simulink model "VFlexP"  (R2025a)
settings: Solver=ode23tb  StartTime=0.0  StopTime=40  FixedStep=5e-5
model workspace (MAT data in the model file):
  DCop_DCBUCK : object (value not decoded)
  Grid_CCVSC_idx = [2; 3; 4; 5; 6; 7; 8; 9; 10; 11; 12]
  Grid_CCVSCs = 1
  Grid_CCVSCs_buses = 1
  Grid_CCVSCs_toM = [0 1 0 0 0 0 0 0 0 0 0 0 ... (781 elements, 71x11)]
  Grid_C_Lines = [0.1 0.1 0.1 0.1]
  Grid_Cbuses = [0.05000002 0.10000002 0.10000002 0.10000002 0.05000002]
  Grid_DC : object (value not decoded)
  Grid_DCop_DCBUCK : object (value not decoded)
  Grid_DCop_DC_PES : object (value not decoded)
  Grid_DFIGs = 1
  Grid_DFIGs_buses = 1
  Grid_DGs : string (value not decoded)
  Grid_From_buses = [1 2 4 4]
  Grid_GFls = 1
  Grid_GFls_buses = 1
  Grid_GFr_idx = [1; 2; 3]
  Grid_GFrs = 1
  Grid_GFrs_buses = 1
  Grid_GFrs_toM = [1 0 0 0 0 0 0 0 0 1 0 0 ... (15 elements, 5x3)]
  Grid_IG_idx = 1
  Grid_IGs = 1
  Grid_IGs_buses = 1
  Grid_IGs_toM = [1; 0]
  Grid_L_Lines = [0.5 0.5 0.5 0.5]
  Grid_L_Loads = [0.000959999944704 0.000156249997559 0.00154855477548]
  Grid_Lines_fromM : object (value not decoded)
  Grid_Lines_toM : object (value not decoded)
  Grid_Load_buses = [2; 3; 4]
  Grid_Load_busesDC = []
  Grid_MGES_idx = [1; 2; 3]
  Grid_MGESs = 1
  Grid_MGESs_buses = [1; 5; 3]
  Grid_MGESs_toM = [1 0 0 0 0 0 0 0 0 1 0 0 ... (15 elements, 5x3)]
  Grid_MSGs = 1
  Grid_MSGs_buses = 1
  Grid_Nbuses = 5
  Grid_PQ_gen = [3; 2; 2]
  Grid_Ploads = [1250 4000 1250]
  Grid_PloadsDC = []
  Grid_Ps_lf = [0.274439537683 0.78 0.3]
  Grid_Qloads = [0.3 0.5 0.5]
  Grid_Qs_lf = [-0.0366071562958 0.126505596722 -0.0162964024532]
  Grid_R_Lines = [0.01 0.01 0.01 0.01]
  Grid_R_Loads = [3.9999997696 1.24999998047 3.8713869387]
  Grid_R_Loads_DC = 0
  Grid_Rcf = [50000000 50000000 50000000 50000000 50000000]
  Grid_SCs = 1
  Grid_SCs_buses = 1
  Grid_SG_idx = 1
  Grid_SGs = 1
  Grid_SGs_buses = 1
  Grid_SGs_toM = [1; 0]
  Grid_To_buses = [2 3 3 5]
  Grid_VCVSC_idx = [1; 2; 3; 4; 5; 6; 7; 8; 9; 10; 11; 12]
  Grid_VCVSCs = 1
  Grid_VCVSCs_buses = [1; 2; 3; 6; 8; 9; 12; 58; 59; 60; 63; 65]
  Grid_VCVSCs_toM = [1 0 0 0 0 0 0 0 0 0 0 0 ... (852 elements, 71x12)]
  Grid_VSM_idx = [1; 2; 3]
  Grid_VSMs = 1
  Grid_VSMs_buses = 1
  Grid_VSMs_toM = [1 0 0 0 0 0 0 0 0 1 0 0 ... (15 elements, 5x3)]
  Grid_admitt_matrix = [2.15353135314-19.7953135314i  -1.9801980198+19.801980198i; -1.9801980198+19.801980198i  2.15353135314-19.7953135314i]
  Grid_admitt_matrix_noloads = [1.98686468647-19.7953135314i  -1.9801980198+19.801980198i; -1.9801980198+19.801980198i  1.98686468647-19.7953135314i]
  Grid_bus = [1; 2; 6; 7; 8]
  Grid_busDC_complexity = [1 1 1]
  Grid_busDC_complexity_PF = [2 2 2]
  Grid_bus_complexity = [1 1 1 1 1]
  Grid_bus_complexity_PF = [1 1 1 1 1]
  Grid_buses_lf = [1; 5; 3]
  Grid_conductance_matrix = [100.00000002  -100  0; -100  200.00000002  -100; 0  -100  100.00000002]
  Grid_conductance_matrix_noloads = [100.00000002  -100  0; -100  200.00000002  -100; 0  -100  100.00000002]
  Grid_fref : object (value not decoded)
  Grid_gen_static_params : mBase (value not decoded)
  Grid_iPs_lf = [3.64378984326 1.28205128205 3.33333333333]
  Grid_iQs_lf = [-27.3170631425 7.90478860943 -61.3632366329]
  Grid_iadmitt_matrix = [2.88165849328-0.0982918688642i  2.87905051706-0.123273862303i; 2.87905051706-0.123273862303i  2.88165849328-0.0982918688642i]
  Grid_iadmitt_matrix_noloads = [37.5012524798-37.4874983544i  37.4987475202-37.5125016456i; 37.4987475202-37.5125016456i  37.5012524798-37.4874983544i]
  Grid_iconductance_matrix = [16666671.4556  16666671.4489  16666671.4456; 16666671.4489  16666671.4522  16666671.4489; 16666671.4456  16666671.4489  16666671.4556]
  Grid_iconductance_matrix_noloads = [16666671.4556  16666671.4489  16666671.4456; 16666671.4489  16666671.4522  16666671.4489; 16666671.4456  16666671.4489  16666671.4556]
  Grid_init_OK_bool = 1
  Grid_intconv_PF : object (value not decoded)
  Grid_lf_op : op_report (value not decoded)
  Grid_lineDC_complexity = [1 1]
  Grid_lineDC_complexity_PF = [2 2]
  Grid_line_complexity = [1 1 1 1]
  Grid_line_complexity_PF = [3 3 3 3]
  Grid_loadDC_complexity = []
  Grid_loadDC_complexity_PF = []
  Grid_load_complexity = [3 3 3]
  Grid_load_complexity_PF = [4 4 4]
  Grid_opDC_CCVSC : object (value not decoded)
  Grid_opDC_VSM : object (value not decoded)
  Grid_opGFr : object (value not decoded)
  Grid_opVCVSC : object (value not decoded)
  Grid_op_CCVSC : object (value not decoded)
  Grid_op_IG : object (value not decoded)
  Grid_op_MGES : object (value not decoded)
  Grid_op_SG : object (value not decoded)
  Grid_op_VSM : object (value not decoded)
  Grid_shift_lines = [0 0 0 0]
  Grid_tap_lines = [1 1 1 1]
  Grid_v_buses_mod = [1 1 1 0.9837920967 1]
  LinsysParamChangeStruct : Param1 (value not decoded)
  Lline = 0.01
  Rline = 1e-05
  linsys : object (value not decoded)
symbols that are objects in the model workspace (value not decoded): Grid_DCop_DC_PES, Grid_DCop_DCBUCK, Grid_op_CCVSC, Grid_op_IG, Grid_op_MGES, Grid_op_SG, Grid_op_VSM, Grid_opDC_CCVSC, Grid_opDC_VSM, Grid_opGFr, Grid_opVCVSC
undefined symbols (not defined in the file): block_buses_DC, block_idx, CCVSC_idx, Cf, costs, costs2, D, DFIGs_nodes, DiscIntNeverNeededParam, entity, Fb, Fi, From_nodes, grid_linsys, Grid_op_DFIG, Grid_op_DFIG_PQ, Grid_op_MSG, Grid_op_SC, Grid_op_VCVSC, H, initial_states_grid, K_1, K_3, K_5, K_A, K_C, K_IM, K_IR, K_P, K_PM, K_PR, K_S1, K_S2, K_S3, Ki_w, Kic, Kiv, Kp_id, Kp_theta, Kp_w, Kpc, Kpv, last_send, Lc, Lf, Lfd, Lkd1, Lkd2, Lkq1, Lkq2, Lkq3, Lmd, Lmq, Lsd, Lsq, m, M, Matrix_flux_to_i, mp, MSGs_buses ... (+44)
libraries: simulink x1048, eeGeneralControl x12
(part 10 of 50)

== system VFlexP/Grid/Generators/DFIG/w_ref_TF ==
  in : Inport
  Gain : Gain  Gain=1/T_s
  Sum4 : Sum  Inputs=|+-
  x_a : Integrator  InitialCondition=Grid_op_DFIG.op.States(23).x'
  out : Outport
  wires:
  Gain/1 -> x_a/1
  Sum4/1 -> Gain/1
  x_a/1 -> out/1, Sum4/2
  in/1 -> Sum4/1

== system VFlexP/Grid/Generators/GFl/CC ==
  note: 1) Add Subsystem or Model blocks as valid variant choices.
      | 2) You cannot connect blocks at this level. At simulation, connectivity is automatically
      | determined, based on the active variant and port name matching.
  idref : Inport
  iqref : Inport  Port=2
  vod : Inport  Port=3
  voq : Inport  Port=4
  omega : Inport  Port=5
  dynamic : Subsystem  VariantControl=dynamic  mask{dynamic_line=Dynamic}
      mask prompts: dynamic_line "Line"
      mask TypeOptions dynamic_line: RL/dynamic
  static : Subsystem  VariantControl=static
  idiref : Outport
  iqiref : Outport  Port=2

== system VFlexP/Grid/Generators/GFl/For Each Subsystem ==
  In1 : Inport  Partition=on  PartitionDimension=1  PartitionWidth=1  PartitionOffset=0
  For Each : ForEach  DisableCoverage=on
  State-Space : StateSpace  A=[]  B=[]  C=[]  D=block_toM  InitialCondition=0  ParameterTunability=Optimized
  Transpose : Math  Operator=transpose
  Transpose1 : Math  Operator=transpose
  Out1 : Outport  ConcatenationDimension=1
  wires:
  Transpose1/1 -> Out1/1
  In1/1 -> Transpose/1
  Transpose/1 -> State-Space/1
  State-Space/1 -> Transpose1/1

== system VFlexP/Grid/Generators/GFl/LPF ==
  In1 : Inport
  Gain : Gain  Gain=1e2
  I : Integrator  InitialCondition=Grid_op_CCVSC.op.States(1).x'
  Sum4 : Sum  Inputs=|+-
  Out1 : Outport
  wires:
  Gain/1 -> I/1
  Sum4/1 -> Gain/1
  In1/1 -> Sum4/1
  I/1 -> Out1/1, Sum4/2

== system VFlexP/Grid/Generators/GFl/LPF1 ==
  In1 : Inport
  Gain : Gain  Gain=1e2
  I : Integrator  InitialCondition=Grid_op_CCVSC.op.States(2).x'
  Sum4 : Sum  Inputs=|+-
  Out1 : Outport
  wires:
  I/1 -> Sum4/2, Out1/1
  In1/1 -> Sum4/1
  Sum4/1 -> Gain/1
  Gain/1 -> I/1

== system VFlexP/Grid/Generators/GFl/LPF2 ==
  In1 : Inport
  Gain : Gain  Gain=1e2
  I : Integrator  InitialCondition=Grid_op_CCVSC.op.States(3).x'
  Sum4 : Sum  Inputs=|+-
  Out1 : Outport
  wires:
  Gain/1 -> I/1
  Sum4/1 -> Gain/1
  In1/1 -> Sum4/1
  I/1 -> Out1/1, Sum4/2

== system VFlexP/Grid/Generators/GFl/LPF3 ==
  In1 : Inport
  Gain : Gain  Gain=1e2
  I : Integrator  InitialCondition=Grid_op_CCVSC.op.States(4).x'
  Sum4 : Sum  Inputs=|+-
  Out1 : Outport
  wires:
  I/1 -> Sum4/2, Out1/1
  In1/1 -> Sum4/1
  Sum4/1 -> Gain/1
  Gain/1 -> I/1

== system VFlexP/Grid/Generators/GFl/LPF_d ==
  In1 : Inport
  Gain : Gain  Gain=iTf
  I : Integrator  InitialCondition=Grid_op_CCVSC.op.States(5).x'
  Sum4 : Sum  Inputs=|+-
  Out1 : Outport
  wires:
  I/1 -> Sum4/2, Out1/1
  In1/1 -> Sum4/1
  Sum4/1 -> Gain/1
  Gain/1 -> I/1

== system VFlexP/Grid/Generators/GFl/LPF_q ==
  In1 : Inport
  Gain : Gain  Gain=iTf
  I : Integrator  InitialCondition=Grid_op_CCVSC.op.States(6).x'
  Sum4 : Sum  Inputs=|+-
  Out1 : Outport
  wires:
  Sum4/1 -> Gain/1
  In1/1 -> Sum4/1
  I/1 -> Sum4/2, Out1/1
  Gain/1 -> I/1

== system VFlexP/Grid/Generators/GFl/PC ==
  vodi : Inport
  voq : Inport  Port=2
  vodi1 : Inport  Port=3
  vodi2 : Inport  Port=4
  omega : Inport  Port=5
  Constant : Constant
  Constant1 : Constant  Value=Eref  VectorParams1D=off
  Constant2 : Constant  Value=Inf
  Divide : Product  Inputs=*/
  Divide1 : Product  Inputs=*/
  Gain1 : Gain  Gain=alphaqcoef
  Gain2 : Gain  Gain=alphapcoef
  LPF_d : Subsystem  Commented=through
  LPF_q : Subsystem  Commented=through
  Product{,1..5} (6 alike) : Product
  Saturation : Subsystem  Commented=through
  Sum : Sum  Inputs=|++
  Sum1 : Sum  Inputs=|+-
  Sum3 : Sum  Inputs=|-+
  Sum4 : Sum  Inputs=|++
  Sum5 : Sum  Inputs=++|
  Sum6 : Sum  Inputs=|-+
  Sum7 : Sum  Inputs=++|
  Switch : Switch  Criteria=u2 > Threshold  Threshold=1e-5  ZeroCross=off  SaturateOnIntegerOverflow=off  InputSameDT=off
  Output : Outport
  Output1 : Outport  Port=2
  wires:
  LPF_q/1(Out1) -> Product5/1, Product5/2, Product2/2, Product1/1
  LPF_d/1(Out1) -> Product4/1, Product4/2, Product/2, Product3/2, Sum6/1
  Switch/1 -> Divide1/2, Divide/2
  Constant2/1 -> Switch/3
  vodi2/1 -> Sum7/2  "Qref"
  Sum6/1 -> Gain1/1
  omega/1 -> Sum3/1  "omega"
  Gain1/1 -> Sum7/1
  Constant1/1 -> Sum6/2
  vodi1/1 -> Sum5/2  "Pref"
  Gain2/1 -> Sum5/1
  Constant/1 -> Sum3/2
  Sum3/1 -> Gain2/1
  Sum/1 -> Divide/1
  Sum4/1 -> Switch/1, Switch/2
  Sum1/1 -> Divide1/1
  Sum5/1 -> Product/1, Product2/1  "Prefnew"
  Product5/1 -> Sum4/2
  Product4/1 -> Sum4/1
  voq/1 -> LPF_q/1(In1)  "voq"
  vodi/1 -> LPF_d/1(In1)  "vod"
  Sum7/1 -> Product3/1, Product1/2  "Qrefnew"
  Product3/1 -> Sum1/2
  Product2/1 -> Sum1/1
  Product1/1 -> Sum/2
  Product/1 -> Sum/1
  Divide/1 -> Saturation/1(ildref)  "ildref"
  Divide1/1 -> Saturation/2(ilqref)  "ilqref"
  Saturation/1(y) -> Output/1
  Saturation/2(y1) -> Output1/1

== system VFlexP/Grid/Generators/GFl/PLL ==
  note: 1) Add Subsystem or Model blocks as valid variant choices.
      | 2) You cannot connect blocks at this level. At simulation, connectivity is automatically
      | determined, based on the active variant and port name matching.
  voutangle : Inport
  vq : Inport  Port=2
  omega : Inport  Port=3
  dynamic : Subsystem  VariantControl=dynamic
  static : Subsystem  VariantControl=static
  theta : Outport
  omega_point : Outport  Port=2

== system VFlexP/Grid/Generators/GFl/Reference frame transform3 ==
  in_d : Inport
  theta : Inport  Port=2
  in_q : Inport  Port=3
  Complex to Real-Imag : ComplexToRealImag
  Cos : Trigonometry  SCDEnableBlockLinearizationSpecification=on  Operator=cos
  Product : Product
  Real-Imag to Complex : RealImagToComplex
  Real-Imag to Complex1 : RealImagToComplex
  Sin : Trigonometry  SCDEnableBlockLinearizationSpecification=on
  out_d : Outport
  out_q : Outport  Port=2
  wires:
  Complex to Real-Imag/2 -> out_q/1
  Real-Imag to Complex1/1 -> Product/1
  Real-Imag to Complex/1 -> Product/2
  Product/1 -> Complex to Real-Imag/1
  theta/1 -> Sin/1, Cos/1
  Cos/1 -> Real-Imag to Complex1/1
  Sin/1 -> Real-Imag to Complex1/2
  Complex to Real-Imag/1 -> out_d/1
  in_q/1 -> Real-Imag to Complex/2
  in_d/1 -> Real-Imag to Complex/1

== system VFlexP/Grid/Generators/GFl/Reference_frame_transform1 ==
  din : Inport
  qin : Inport  Port=2
  theta : Inport  Port=3
  Complex to Real-Imag : ComplexToRealImag
  Cos : Trigonometry  SCDEnableBlockLinearizationSpecification=on  Operator=cos
  Product : Product
  Real-Imag to Complex : RealImagToComplex
  Real-Imag to Complex1 : RealImagToComplex
  Sin : Trigonometry  SCDEnableBlockLinearizationSpecification=on
  dout : Outport
  qout : Outport  Port=2
  wires:
  Sin/1 -> Real-Imag to Complex1/2
  Cos/1 -> Real-Imag to Complex1/1
  theta/1 -> Cos/1, Sin/1
  Product/1 -> Complex to Real-Imag/1
  Real-Imag to Complex/1 -> Product/2
  qin/1 -> Real-Imag to Complex/2
  din/1 -> Real-Imag to Complex/1
  Real-Imag to Complex1/1 -> Product/1
  Complex to Real-Imag/2 -> qout/1
  Complex to Real-Imag/1 -> dout/1

== system VFlexP/Grid/Generators/GFl/connect ==
  id : Inport
  iq : Inport  Port=2
  connect : Inport  Port=3
  Switch : Switch  Criteria=u2 > Threshold  ZeroCross=off  SaturateOnIntegerOverflow=off  InputSameDT=off
  Switch1 : Switch  Criteria=u2 > Threshold  ZeroCross=off  SaturateOnIntegerOverflow=off  InputSameDT=off
  Zero1 : Constant  Value=0  VectorParams1D=off  OutDataTypeStr=Inherit: Inherit via back propagation
  Zero2 : Constant  Value=0  VectorParams1D=off  OutDataTypeStr=Inherit: Inherit via back propagation
  id_real : Outport
  iq_real : Outport  Port=2
  connected : Outport  Port=3  OutDataTypeStr=boolean
  wires:
  Switch/1 -> id_real/1
  Zero1/1 -> Switch/3
  id/1 -> Switch/1
  connect/1 -> connected/1, Switch1/2, Switch/2
  Switch1/1 -> iq_real/1
  iq/1 -> Switch1/1
  Zero2/1 -> Switch1/3

== system VFlexP/Grid/Generators/GFl/trim_output ==
  id : Inport
  iq : Inport  Port=2
  vd : Inport  Port=3
  vq : Inport  Port=4
  Out1 : Outport
  Out2 : Outport  Port=2
  Out3 : Outport  Port=3
  Out4 : Outport  Port=4
  wires:
  id/1 -> Out1/1
  vq/1 -> Out4/1
  vd/1 -> Out3/1
  iq/1 -> Out2/1

== system VFlexP/Grid/Generators/GFr/For Each Subsystem ==
  In1 : Inport  Partition=on  PartitionDimension=1  PartitionWidth=1  PartitionOffset=0
  For Each : ForEach  DisableCoverage=on
  State-Space : StateSpace  A=[]  B=[]  C=[]  D=block_toM  InitialCondition=0  ParameterTunability=Optimized
  Transpose : Math  Operator=transpose
  Transpose1 : Math  Operator=transpose
  Out1 : Outport  ConcatenationDimension=1
  wires:
  In1/1 -> Transpose/1
  State-Space/1 -> Transpose1/1
  Transpose/1 -> State-Space/1
  Transpose1/1 -> Out1/1

== system VFlexP/Grid/Generators/GFr/LPF ==
  In1 : Inport
  Gain : Gain  Gain=1e2
  I : Integrator  InitialCondition=Grid_op_VCVSC.op.States(4).x'
  Sum4 : Sum  Inputs=|+-
  Out1 : Outport
  wires:
  Gain/1 -> I/1
  Sum4/1 -> Gain/1
  In1/1 -> Sum4/1
  I/1 -> Out1/1, Sum4/2

== system VFlexP/Grid/Generators/GFr/LPF1 ==
  In1 : Inport
  Gain : Gain  Gain=1e2
  I : Integrator  InitialCondition=Grid_op_VCVSC.op.States(5).x'
  Sum4 : Sum  Inputs=|+-
  Out1 : Outport
  wires:
  I/1 -> Sum4/2, Out1/1
  In1/1 -> Sum4/1
  Sum4/1 -> Gain/1
  Gain/1 -> I/1

== system VFlexP/Grid/Generators/GFr/LPF_P ==
  P : Inport
  Gain : Gain  Gain=100
  I : Integrator  InitialCondition=Grid_opGFr.Pd
  Sum4 : Sum  Inputs=|+-
  P_f : Outport
  wires:
  Gain/1 -> I/1
  Sum4/1 -> Gain/1
  P/1 -> Sum4/1
  I/1 -> P_f/1, Sum4/2

== system VFlexP/Grid/Generators/GFr/LPF_omega ==
  in : Inport
  Gain : Gain  Gain=100
  I : Integrator  InitialCondition=1
  Sum4 : Sum  Inputs=|+-
  out : Outport
  wires:
  Gain/1 -> I/1
  Sum4/1 -> Gain/1
  in/1 -> Sum4/1
  I/1 -> Sum4/2, out/1

== system VFlexP/Grid/Generators/GFr/LPF_v ==
  in : Inport
  Gain : Gain  Gain=100
  I : Integrator  InitialCondition=Grid_opGFr.v
  Sum4 : Sum  Inputs=|+-
  out : Outport
  wires:
  Gain/1 -> I/1
  Sum4/1 -> Gain/1
  in/1 -> Sum4/1
  I/1 -> Sum4/2, out/1

== system VFlexP/Grid/Generators/GFr/PC ==
  ioq : Inport
  iodi : Inport  Port=2
  omegaref : Inport  Port=3
  Eref : Inport  Port=4
  vodi : Inport  Port=5
  voq : Inport  Port=6
  Psp : Inport  Port=7
  Qsp : Inport  Port=8
  LPF_P : Subsystem
  LPF_Q : Subsystem
  Product{,1..3} (4 alike) : Product
  Sum : Sum  Inputs=|++
  Sum1 : Sum  Inputs=|-+
  Sum2 : Sum  Inputs=|+-
  Sum3 : Sum  Inputs=|-+
  Sum4 : Sum  Inputs=|+-
  Sum5 : Sum  Inputs=-+|
  mp1 : Gain  Gain=mp
  nq1 : Gain  Gain=nq
  Out1 : Outport
  Out2 : Outport  Port=2
  P_f : Outport  Port=3
  Q_f : Outport  Port=4
  wires:
  Sum2/1 -> Out1/1  "omega"
  vodi/1 -> Product2/1, Product/1  "vod"
  Product/1 -> Sum/1
  Product1/1 -> Sum/2
  Product2/1 -> Sum1/1
  Product3/1 -> Sum1/2
  nq1/1 -> Sum3/1  "nqQ"
  Eref/1 -> Sum3/2  "Eref"
  omegaref/1 -> Sum2/1  "omegaref"
  Sum/1 -> Sum5/2, P_f/1
  Sum1/1 -> Q_f/1, Sum4/1
  mp1/1 -> Sum2/2  "mpP"
  voq/1 -> Product1/1, Product3/1  "voq"
  iodi/1 -> Product3/2, Product/2  "iod"
  ioq/1 -> Product2/2, Product1/2  "ioq"
  Qsp/1 -> Sum4/2
  Sum4/1 -> LPF_Q/1(Q)
  Sum5/1 -> LPF_P/1(P)
  Sum3/1 -> Out2/1  "vodref"
  LPF_P/1(P_f) -> mp1/1
  LPF_Q/1(Q_f) -> nq1/1
  Psp/1 -> Sum5/1

== system VFlexP/Grid/Generators/GFr/PI_synchro_f ==
  In1 : Inport
  Gain : Gain  Gain=0.1
  Gain1 : Gain  Gain=0.2
  I : Integrator
  Sum10 : Sum  Inputs=|++
  Out1 : Outport
  wires:
  Sum10/1 -> Out1/1
  Gain/1 -> Sum10/1
  I/1 -> Sum10/2
  Gain1/1 -> I/1
  In1/1 -> Gain/1, Gain1/1

== system VFlexP/Grid/Generators/GFr/PI_synchro_v ==
  In1 : Inport
  Gain : Gain  Gain=0.1
  Gain1 : Gain  Gain=0.2
  Gain2 : Gain  Gain=5
  I : Integrator
  Sum10 : Sum  Inputs=|++
  Out1 : Outport
  wires:
  Gain1/1 -> I/1
  I/1 -> Sum10/2
  Gain/1 -> Sum10/1
  Sum10/1 -> Out1/1
  In1/1 -> Gain2/1
  Gain2/1 -> Gain/1, Gain1/1

== system VFlexP/Grid/Generators/GFr/RL out ==
  note: 1) Add Subsystem or Model blocks as valid variant choices.
      | 2) You cannot connect blocks at this level. At simulation, connectivity is automatically
      | determined, based on the active variant and port name matching.
  v_in_d : Inport
  v_out_d : Inport  Port=2
  v_in_q : Inport  Port=3
  v_out_q : Inport  Port=4
  dynamic : Subsystem  VariantControl=dynamic
  static : Subsystem  VariantControl=static
  static_omega : Subsystem  VariantControl=static_omega
  id : Outport
  iq : Outport  Port=2
  v_outd : Outport  Port=3
  v_outq : Outport  Port=4

== system VFlexP/Grid/Generators/GFr/Reference frame transform1 ==
  in_d : Inport
  theta : Inport  Port=2
  in_q : Inport  Port=3
  Complex to Real-Imag : ComplexToRealImag
  Cos : Trigonometry  SCDEnableBlockLinearizationSpecification=on  Operator=cos
  Product : Product
  Real-Imag to Complex : RealImagToComplex
  Real-Imag to Complex1 : RealImagToComplex
  Sin : Trigonometry  SCDEnableBlockLinearizationSpecification=on
  out_d : Outport
  out_q : Outport  Port=2
  wires:
  Complex to Real-Imag/2 -> out_q/1
  Real-Imag to Complex1/1 -> Product/1
  Real-Imag to Complex/1 -> Product/2
  Product/1 -> Complex to Real-Imag/1
  theta/1 -> Sin/1, Cos/1
  Cos/1 -> Real-Imag to Complex1/1
  Sin/1 -> Real-Imag to Complex1/2
  Complex to Real-Imag/1 -> out_d/1
  in_q/1 -> Real-Imag to Complex/2
  in_d/1 -> Real-Imag to Complex/1

== system VFlexP/Grid/Generators/GFr/Reference frame transform2 ==
  in_d : Inport
  theta : Inport  Port=2
  in_q : Inport  Port=3
  Complex to Real-Imag : ComplexToRealImag
  Cos : Trigonometry  SCDEnableBlockLinearizationSpecification=on  Operator=cos
  Product : Product
  Real-Imag to Complex : RealImagToComplex
  Real-Imag to Complex1 : RealImagToComplex
  Sin : Trigonometry  SCDEnableBlockLinearizationSpecification=on
  out_d : Outport
  out_q : Outport  Port=2
  wires:
  in_d/1 -> Real-Imag to Complex/1
  in_q/1 -> Real-Imag to Complex/2
  Complex to Real-Imag/1 -> out_d/1
  Sin/1 -> Real-Imag to Complex1/2
  Cos/1 -> Real-Imag to Complex1/1
  theta/1 -> Cos/1, Sin/1
  Product/1 -> Complex to Real-Imag/1
  Real-Imag to Complex/1 -> Product/2
  Real-Imag to Complex1/1 -> Product/1
  Complex to Real-Imag/2 -> out_q/1

== system VFlexP/Grid/Generators/GFr/Reference frame transform3 ==
  in_d : Inport
  theta : Inport  Port=2
  in_q : Inport  Port=3
  Complex to Real-Imag : ComplexToRealImag
  Cos : Trigonometry  SCDEnableBlockLinearizationSpecification=on  Operator=cos
  Product : Product
  Real-Imag to Complex : RealImagToComplex
  Real-Imag to Complex1 : RealImagToComplex
  Sin : Trigonometry  SCDEnableBlockLinearizationSpecification=on
  out_d : Outport
  out_q : Outport  Port=2
  wires:
  Complex to Real-Imag/2 -> out_q/1
  Real-Imag to Complex1/1 -> Product/1
  Real-Imag to Complex/1 -> Product/2
  Product/1 -> Complex to Real-Imag/1
  theta/1 -> Cos/1, Sin/1
  Cos/1 -> Real-Imag to Complex1/1
  Sin/1 -> Real-Imag to Complex1/2
  Complex to Real-Imag/1 -> out_d/1
  in_q/1 -> Real-Imag to Complex/2
  in_d/1 -> Real-Imag to Complex/1

== system VFlexP/Grid/Generators/GFr/VCC ==
  note: 1) Add Subsystem or Model blocks as valid variant choices.
      | 2) You cannot connect blocks at this level. At simulation, connectivity is automatically
      | determined, based on the active variant and port name matching.
  vodref : Inport
  voqref : Inport  Port=2
  iod : Inport  Port=3
  ioq : Inport  Port=4
  omega : Inport  Port=5
  dynamic : Subsystem  VariantControl=dynamic
  dynamic_VC : Subsystem  VariantControl=dynamic_VC
  dynamic_limiting : Subsystem  VariantControl=dynamic_limiting
  static : Subsystem  VariantControl=static
  vidref : Outport
  viqref : Outport  Port=2

== system VFlexP/Grid/Generators/GFr/VI ==
  id : Inport
  iq : Inport  Port=2
  omega : Inport  Port=3
  Gain : Gain  Gain=L
  Gain1 : Gain  Gain=R
  Gain2 : Gain  Gain=L
  Gain3 : Gain  Gain=R
  Product : Product
  Product1 : Product
  Sum : Sum  Inputs=-+|
  Sum1 : Sum  Inputs=|--
  WOF_d : Subsystem  Commented=through
  WOF_q : Subsystem  Commented=through
  vd : Outport
  vq : Outport  Port=2
  wires:
  WOF_q/1(Out1) -> Gain/1, Gain3/1
  WOF_d/1(Out1) -> Gain1/1, Gain2/1
  Sum1/1 -> vq/1
  Sum/1 -> vd/1
  Gain3/1 -> Sum1/2
  Gain1/1 -> Sum/1
  Product1/1 -> Sum1/1
  Gain2/1 -> Product1/2
  id/1 -> WOF_d/1(In1)
  Product/1 -> Sum/2
  iq/1 -> WOF_q/1(In1)
  omega/1 -> Product1/1, Product/2
  Gain/1 -> Product/1

== system VFlexP/Grid/Generators/GFr/connect ==
  id : Inport
  iq : Inport  Port=2
  connect : Inport  Port=3
  Switch : Switch  Criteria=u2 > Threshold  ZeroCross=off  SaturateOnIntegerOverflow=off  InputSameDT=off
  Switch1 : Switch  Criteria=u2 > Threshold  ZeroCross=off  SaturateOnIntegerOverflow=off  InputSameDT=off
  Zero1 : Constant  Value=0  VectorParams1D=off  OutDataTypeStr=Inherit: Inherit via back propagation
  Zero2 : Constant  Value=0  VectorParams1D=off  OutDataTypeStr=Inherit: Inherit via back propagation
  id_real : Outport
  iq_real : Outport  Port=2
  connected : Outport  Port=3  OutDataTypeStr=boolean
  wires:
  Switch/1 -> id_real/1
  Zero1/1 -> Switch/3
  id/1 -> Switch/1
  connect/1 -> connected/1, Switch1/2, Switch/2
  Switch1/1 -> iq_real/1
  iq/1 -> Switch1/1
  Zero2/1 -> Switch1/3

== system VFlexP/Grid/Generators/GFr/trim_output ==
  id : Inport
  iq : Inport  Port=2
  vd : Inport  Port=3
  vq : Inport  Port=4
  Out1 : Outport
  Out2 : Outport  Port=2
  Out3 : Outport  Port=3
  Out4 : Outport  Port=4
  wires:
  id/1 -> Out1/1
  vq/1 -> Out4/1
  vd/1 -> Out3/1
  iq/1 -> Out2/1

== system VFlexP/Grid/Generators/IG/For Each Subsystem ==
  In1 : Inport  Partition=on  PartitionDimension=1  PartitionWidth=1  PartitionOffset=0
  For Each : ForEach  DisableCoverage=on
  State-Space : StateSpace  A=[]  B=[]  C=[]  D=block_toM  InitialCondition=0  ParameterTunability=Optimized
  Transpose : Math  Operator=transpose
  Transpose1 : Math  Operator=transpose
  Out1 : Outport  ConcatenationDimension=1
  wires:
  Transpose1/1 -> Out1/1
  In1/1 -> Transpose/1
  Transpose/1 -> State-Space/1
  State-Space/1 -> Transpose1/1

== system VFlexP/Grid/Generators/IG/PQ ==
  vd : Inport
  id : Inport  Port=2
  vq : Inport  Port=3
  iq : Inport  Port=4
  LPF_P : Subsystem
  LPF_Q : Subsystem
  Product{,1..3} (4 alike) : Product
  Sum : Sum  Inputs=|++
  Sum1 : Sum  Inputs=|+-
  P : Outport
  Q : Outport  Port=2
  wires:
  Product/1 -> Sum/1
  Sum/1 -> LPF_P/1(P)
  vd/1 -> Product3/1, Product/1
  id/1 -> Product2/2, Product/2
  vq/1 -> Product2/1, Product1/1
  iq/1 -> Product3/2, Product1/2
  Product1/1 -> Sum/2
  Sum1/1 -> LPF_Q/1(Q)
  Product2/1 -> Sum1/1
  Product3/1 -> Sum1/2
  LPF_P/1(P_f) -> P/1
  LPF_Q/1(Q_f) -> Q/1

== system VFlexP/Grid/Generators/IG/RL out ==
  note: 1) Add Subsystem or Model blocks as valid variant choices.
      | 2) You cannot connect blocks at this level. At simulation, connectivity is automatically
      | determined, based on the active variant and port name matching.
  v_in_d : Inport
  v_out_d : Inport  Port=2
  v_in_q : Inport  Port=3
  v_out_q : Inport  Port=4
  dynamic : Subsystem  VariantControl=dynamic
  static : Subsystem  VariantControl=static
  static_omega : Subsystem  VariantControl=static_omega
  id : Outport
  iq : Outport  Port=2
  v_outd : Outport  Port=3
  v_outq : Outport  Port=4

== system VFlexP/Grid/Generators/IG/Reference frame transform2 ==
  in_d : Inport
  theta : Inport  Port=2
  in_q : Inport  Port=3
  Complex to Real-Imag : ComplexToRealImag
  Cos : Trigonometry  SCDEnableBlockLinearizationSpecification=on  Operator=cos
  Product : Product
  Real-Imag to Complex : RealImagToComplex
  Real-Imag to Complex1 : RealImagToComplex
  Sin : Trigonometry  SCDEnableBlockLinearizationSpecification=on
  out_d : Outport
  out_q : Outport  Port=2
  wires:
  in_d/1 -> Real-Imag to Complex/1
  in_q/1 -> Real-Imag to Complex/2
  Complex to Real-Imag/1 -> out_d/1
  Sin/1 -> Real-Imag to Complex1/2
  Cos/1 -> Real-Imag to Complex1/1
  theta/1 -> Cos/1, Sin/1
  Product/1 -> Complex to Real-Imag/1
  Real-Imag to Complex/1 -> Product/2
  Real-Imag to Complex1/1 -> Product/1
  Complex to Real-Imag/2 -> out_q/1

== system VFlexP/Grid/Generators/IG/connect ==
  id : Inport
  iq : Inport  Port=2
  connect : Inport  Port=3
  Switch : Switch  Criteria=u2 > Threshold  ZeroCross=off  SaturateOnIntegerOverflow=off  InputSameDT=off
  Switch1 : Switch  Criteria=u2 > Threshold  ZeroCross=off  SaturateOnIntegerOverflow=off  InputSameDT=off
  Zero1 : Constant  Value=0  VectorParams1D=off  OutDataTypeStr=Inherit: Inherit via back propagation
  Zero2 : Constant  Value=0  VectorParams1D=off  OutDataTypeStr=Inherit: Inherit via back propagation
  id_real : Outport
  iq_real : Outport  Port=2
  connected : Outport  Port=3  OutDataTypeStr=boolean
  wires:
  Switch/1 -> id_real/1
  Zero1/1 -> Switch/3
  id/1 -> Switch/1
  connect/1 -> connected/1, Switch1/2, Switch/2
  Switch1/1 -> iq_real/1
  iq/1 -> Switch1/1
  Zero2/1 -> Switch1/3

== system VFlexP/Grid/Generators/IG/trim_output ==
  id : Inport
  iq : Inport  Port=2
  vd : Inport  Port=3
  vq : Inport  Port=4
  Out1 : Outport
  Out2 : Outport  Port=2
  Out3 : Outport  Port=3
  Out4 : Outport  Port=4
  wires:
  id/1 -> Out1/1
  vq/1 -> Out4/1
  vd/1 -> Out3/1
  iq/1 -> Out2/1

== system VFlexP/Grid/Generators/MGES/AVR_Exciter ==
  in : Inport
  Gain : Gain  Gain=1./T_s
  Sum4 : Sum  Inputs=|+-
  x_a : Integrator  InitialCondition=Grid_op_MGES.op.States(1).x'
  out : Outport
  wires:
  Gain/1 -> x_a/1
  Sum4/1 -> Gain/1
  in/1 -> Sum4/1
  x_a/1 -> out/1, Sum4/2

== system VFlexP/Grid/Generators/MGES/AVR_Vmeas_Filter ==
  in : Inport
  Gain : Gain  Gain=1./T_r
  Sum4 : Sum  Inputs=|+-
  x_a : Integrator  InitialCondition=Grid_op_MGES.op.States(2).x'
  out : Outport
  wires:
  Gain/1 -> x_a/1
  Sum4/1 -> Gain/1
  in/1 -> Sum4/1
  x_a/1 -> out/1, Sum4/2

== system VFlexP/Grid/Generators/MGES/AVR_Vmeas_Filter1 ==
  in : Inport
  Gain : Gain  Gain=1/T_r
  Sum4 : Sum  Inputs=|+-
  x_a : Integrator  InitialConditionSource=external  InitialCondition=Grid_op_MGES.op.States(3).x'
  out : Outport
  wires:
  x_a/1 -> Sum4/2, out/1
  in/1 -> x_a/2, Sum4/1
  Sum4/1 -> Gain/1
  Gain/1 -> x_a/1

== system VFlexP/Grid/Generators/MGES/AVR_Vmeas_Filter2 ==
  in : Inport
  Gain : Gain  Gain=1/T_r
  Sum4 : Sum  Inputs=|+-
  x_a : Integrator  InitialCondition=Grid_op_SG.op.States(5).x'
  out : Outport
  wires:
  Gain/1 -> x_a/1
  Sum4/1 -> Gain/1
  in/1 -> Sum4/1
  x_a/1 -> out/1, Sum4/2

== system VFlexP/Grid/Generators/MGES/AVR_Vmeas_Filter3 ==
  in : Inport
  Gain : Gain  Gain=1./T_r
  Sum4 : Sum  Inputs=|+-
  x_a : Integrator  InitialCondition=Grid_op_MGES.op.States(4).x'
  out : Outport
  wires:
  x_a/1 -> Sum4/2, out/1
  in/1 -> Sum4/1
  Sum4/1 -> Gain/1
  Gain/1 -> x_a/1

== system VFlexP/Grid/Generators/MGES/Electromagnetic ==
  note: 1) Add Subsystem or Model blocks as valid variant choices.
      | 2) You cannot connect blocks at this level. At simulation, connectivity is automatically
      | determined, based on the active variant and port name matching.
  vsd : Inport
  vsq : Inport  Port=2
  vfd : Inport  Port=3
  ws : Inport  Port=4
  order 2 : Subsystem  VariantControl=order 2
  order 8 : Subsystem  VariantControl=order 8
  order 8 nomatrix : Subsystem  VariantControl=order 1  mask{Lssd_pu=Lssd_pu, Lssq_pu=Lssq_pu, Lmd_pu=Lmd_pu, Lmq_pu=Lmq_pu, Lfd_pu=Lfd_pu, Lkd1_pu=Lkd1_pu, Lkd2_pu=Lkd2_pu, Lkq1_pu=Lkq1_pu, Lkq2_pu=Lkq2_pu, Lkq3_pu=Lkq3_pu}
      mask init:
      | for i=1:length(Lssd_pu)
      |         Lssd = Lssd_pu;
      |         Lssq = Lssq_pu;
      |         Lmd = Lmd_pu;
      |         Lmq = Lmq_pu;
      |         Lfd = Lfd_pu;
      |         Lkd1 = Lkd1_pu;
      |         Lkd2 = Lkd2_pu;
      |         Lkq1 = Lkq1_pu;
      |         Lkq2 = Lkq2_pu;
      |         Lkq3 = Lkq3_pu;
      |         Matrix_flux_to_i(:,:,i) = [(0 - (Lfd(i)*Lmd(i)^2 + Lkd2(i)*Lmd(i)^2 - Lmd(i)^3 - Lfd(i)*Lkd1(i)*Lkd2(i))/(2*Lmd(i)^4 - Lkd1(i)*Lmd(i)^3 - 2*Lkd2(i)*Lmd(i)^3 - Lmd(i)^3*Lssd(i) - 2*Lfd(i)*Lmd(i)^3 + Lfd(i)*Lkd1(i)*Lmd(i)^2 + Lfd(i)*Lkd2(i)*Lmd(i)^2 + Lkd1(i)*Lkd2(i)*Lmd(i)^2 + Lfd(i)*Lmd(i)^2*Lssd(i) + Lkd2(i)*Lmd(i)^2*Lssd(i) - Lfd(i)*Lkd1(i)*Lkd2(i)*Lssd(i))),  + 0,  + (0 + (Lkd1(i)*Lmd(i)^2 + Lkd2(i)*Lmd(i)^2 - Lmd(i)^3 - Lkd1(i)*Lkd2(i)*Lmd(i))/(2*Lmd(i)^4 - Lkd1(i)*Lmd(i)^3 - 2*Lkd2(i)*Lmd(i)^3 - Lmd(i)^3*Lssd(i) - 2*Lfd(i)*Lmd(i)^3 + Lfd(i)*Lkd1(i)*Lmd(i)^2 + Lfd(i)*Lkd2(i)*Lmd(i)^2 + Lkd1(i)*Lkd2(i)*Lmd(i)^2 + Lfd(i)*Lmd(i)^2*Lssd(i) + Lkd2(i)*Lmd(i)^2*Lssd(i) - Lfd(i)*Lkd1(i)*Lkd2(i)*Lssd(i))),  + (0 + (Lfd(i)*Lmd(i)^2 + Lkd2(i)*Lmd(i)^2 - Lmd(i)^3 - Lfd(i)*Lkd2(i)*Lmd(i))/(2*Lmd(i)^4 - Lkd1(i)*Lmd(i)^3 - 2*Lkd2(i)*Lmd(i)^3 - Lmd(i)^3*Lssd(i) - 2*Lfd(i)*Lmd(i)^3 + Lfd(i)*Lkd1(i)*Lmd(i)^2 + Lfd(i)*Lkd2(i)*Lmd(i)^2 + Lkd1(i)*Lkd2(i)*Lmd(i)^2 + Lfd(i)*Lmd(i)^2*Lssd(i) + Lkd2(i)*Lmd(i)^2*Lssd(i) - Lfd(i)*Lkd1(i)*Lkd2(i)*Lssd(i))),  + (0 + (Lfd(i)*Lmd(i)^2 - Lfd(i)*Lkd1(i)*Lmd(i))/(2*Lmd(i)^4 - Lkd1(i)*Lmd(i)^3 - 2*Lkd2(i)*Lmd(i)^3 - Lmd(i)^3*Lssd(i) - 2*Lfd(i)*Lmd(i)^3 + Lfd(i)*Lkd1(i)*Lmd(i)^2 + Lfd(i)*Lkd2(i)*Lmd(i)^2 + Lkd1(i)*Lkd2(i)*Lmd(i)^2 + Lfd(i)*Lmd(i)^2*Lssd(i) + Lkd2(i)*Lmd(i)^2*Lssd(i) - Lfd(i)*Lkd1(i)*Lkd2(i)*Lssd(i))),  + 0,  + 0,  + 0, ; 0,  + (0 - (Lkq1(i)*Lmq(i)^2 + Lkq2(i)*Lmq(i)^2 + Lkq3(i)*Lmq(i)^2 - 2*Lmq(i)^3 - Lkq1(i)*Lkq2(i)*Lkq3(i))/(3*Lmq(i)^4 - 2*Lkq2(i)*Lmq(i)^3 - 2*Lkq3(i)*Lmq(i)^3 - 2*Lmq(i)^3*Lssq(i) - 2*Lkq1(i)*Lmq(i)^3 + Lkq1(i)*Lkq2(i)*Lmq(i)^2 + Lkq1(i)*Lkq3(i)*Lmq(i)^2 + Lkq2(i)*Lkq3(i)*Lmq(i)^2 + Lkq1(i)*Lmq(i)^2*Lssq(i) + Lkq2(i)*Lmq(i)^2*Lssq(i) + Lkq3(i)*Lmq(i)^2*Lssq(i) - Lkq1(i)*Lkq2(i)*Lkq3(i)*Lssq(i))),  + 0,  + 0,  + 0,  + (0 - (3*Lmq(i)^3 - 2*Lkq2(i)*Lmq(i)^2 - 2*Lkq3(i)*Lmq(i)^2 - 2*Lkq1(i)*Lmq(i)^2 + Lkq1(i)*Lkq2(i)*Lmq(i) + Lkq1(i)*Lkq3(i)*Lmq(i) + Lkq2(i)*Lkq3(i)*Lmq(i))/(3*Lmq(i)^4 - 2*Lkq2(i)*Lmq(i)^3 - 2*Lkq3(i)*Lmq(i)^3 - 2*Lmq(i)^3*Lssq(i) - 2*Lkq1(i)*Lmq(i)^3 + Lkq1(i)*Lkq2(i)*Lmq(i)^2 + Lkq1(i)*Lkq3(i)*Lmq(i)^2 + Lkq2(i)*Lkq3(i)*Lmq(i)^2 + Lkq1(i)*Lmq(i)^2*Lssq(i) + Lkq2(i)*Lmq(i)^2*Lssq(i) + Lkq3(i)*Lmq(i)^2*Lssq(i) - Lkq1(i)*Lkq2(i)*Lkq3(i)*Lssq(i))),  + 0,  + 0, ; (0 - (Lkd2(i)*Lmd(i)^2 - Lkd1(i)*Lkd2(i)*Lmd(i))/(2*Lmd(i)^4 - Lkd1(i)*Lmd(i)^3 - 2*Lkd2(i)*Lmd(i)^3 - Lmd(i)^3*Lssd(i) - 2*Lfd(i)*Lmd(i)^3 + Lfd(i)*Lkd1(i)*Lmd(i)^2 + Lfd(i)*Lkd2(i)*Lmd(i)^2 + Lkd1(i)*Lkd2(i)*Lmd(i)^2 + Lfd(i)*Lmd(i)^2*Lssd(i) + Lkd2(i)*Lmd(i)^2*Lssd(i) - Lfd(i)*Lkd1(i)*Lkd2(i)*Lssd(i))),  + 0,  + (0 + (Lkd1(i)*Lmd(i)^2 + Lkd2(i)*Lmd(i)^2 + Lmd(i)^2*Lssd(i) - 2*Lmd(i)^3 - Lkd1(i)*Lkd2(i)*Lssd(i))/(2*Lmd(i)^4 - Lkd1(i)*Lmd(i)^3 - 2*Lkd2(i)*Lmd(i)^3 - Lmd(i)^3*Lssd(i) - 2*Lfd(i)*Lmd(i)^3 + Lfd(i)*Lkd1(i)*Lmd(i)^2 + Lfd(i)*Lkd2(i)*Lmd(i)^2 + Lkd1(i)*Lkd2(i)*Lmd(i)^2 + Lfd(i)*Lmd(i)^2*Lssd(i) + Lkd2(i)*Lmd(i)^2*Lssd(i) - Lfd(i)*Lkd1(i)*Lkd2(i)*Lssd(i))),  + (0 - (Lkd2(i)*Lmd(i)^2 - Lkd2(i)*Lssd(i)*Lmd(i))/(2*Lmd(i)^4 - Lkd1(i)*Lmd(i)^3 - 2*Lkd2(i)*Lmd(i)^3 - Lmd(i)^3*Lssd(i) - 2*Lfd(i)*Lmd(i)^3 + Lfd(i)*Lkd1(i)*Lmd(i)^2 + Lfd(i)*Lkd2(i)*Lmd(i)^2 + Lkd1(i)*Lkd2(i)*Lmd(i)^2 + Lfd(i)*Lmd(i)^2*Lssd(i) + Lkd2(i)*Lmd(i)^2*Lssd(i) - Lfd(i)*Lkd1(i)*Lkd2(i)*Lssd(i))),  + (0 - (Lkd1(i)*Lmd(i)^2 + Lmd(i)^2*Lssd(i) - 2*Lmd(i)^3)/(2*Lmd(i)^4 - Lkd1(i)*Lmd(i)^3 - 2*Lkd2(i)*Lmd(i)^3 - Lmd(i)^3*Lssd(i) - 2*Lfd(i)*Lmd(i)^3 + Lfd(i)*Lkd1(i)*Lmd(i)^2 + Lfd(i)*Lkd2(i)*Lmd(i)^2 + Lkd1(i)*Lkd2(i)*Lmd(i)^2 + Lfd(i)*Lmd(i)^2*Lssd(i) + Lkd2(i)*Lmd(i)^2*Lssd(i) - Lfd(i)*Lkd1(i)*Lkd2(i)*Lssd(i))),  + 0,  + 0,  + 0, ; (0 - (Lfd(i)*Lmd(i)^2 + Lkd2(i)*Lmd(i)^2 - Lmd(i)^3 - Lfd(i)*Lkd2(i)*Lmd(i))/(2*Lmd(i)^4 - Lkd1(i)*Lmd(i)^3 - 2*Lkd2(i)*Lmd(i)^3 - Lmd(i)^3*Lssd(i) - 2*Lfd(i)*Lmd(i)^3 + Lfd(i)*Lkd1(i)*Lmd(i)^2 + Lfd(i)*Lkd2(i)*Lmd(i)^2 + Lkd1(i)*Lkd2(i)*Lmd(i)^2 + Lfd(i)*Lmd(i)^2*Lssd(i) + Lkd2(i)*Lmd(i)^2*Lssd(i) - Lfd(i)*Lkd1(i)*Lkd2(i)*Lssd(i))),  + 0,  + (0 - (Lkd2(i)*Lmd(i)^2 + Lmd(i)^2*Lssd(i) - Lmd(i)^3 - Lkd2(i)*Lmd(i)*Lssd(i))/(2*Lmd(i)^4 - Lkd1(i)*Lmd(i)^3 - 2*Lkd2(i)*Lmd(i)^3 - Lmd(i)^3*Lssd(i) - 2*Lfd(i)*Lmd(i)^3 + Lfd(i)*Lkd1(i)*Lmd(i)^2 + Lfd(i)*Lkd2(i)*Lmd(i)^2 + Lkd1(i)*Lkd2(i)*Lmd(i)^2 + Lfd(i)*Lmd(i)^2*Lssd(i) + Lkd2(i)*Lmd(i)^2*Lssd(i) - Lfd(i)*Lkd1(i)*Lkd2(i)*Lssd(i))),  + (0 + (Lfd(i)*Lmd(i)^2 + Lkd2(i)*Lmd(i)^2 - Lmd(i)^3 - Lfd(i)*Lkd2(i)*Lssd(i))/(2*Lmd(i)^4 - Lkd1(i)*Lmd(i)^3 - 2*Lkd2(i)*Lmd(i)^3 - Lmd(i)^3*Lssd(i) - 2*Lfd(i)*Lmd(i)^3 + Lfd(i)*Lkd1(i)*Lmd(i)^2 + Lfd(i)*Lkd2(i)*Lmd(i)^2 + Lkd1(i)*Lkd2(i)*Lmd(i)^2 + Lfd(i)*Lmd(i)^2*Lssd(i) + Lkd2(i)*Lmd(i)^2*Lssd(i) - Lfd(i)*Lkd1(i)*Lkd2(i)*Lssd(i))),  + (0 - (Lfd(i)*Lmd(i)^2 - Lfd(i)*Lssd(i)*Lmd(i))/(2*Lmd(i)^4 - Lkd1(i)*Lmd(i)^3 - 2*Lkd2(i)*Lmd(i)^3 - Lmd(i)^3*Lssd(i) - 2*Lfd(i)*Lmd(i)^3 + Lfd(i)*Lkd1(i)*Lmd(i)^2 + Lfd(i)*Lkd2(i)*Lmd(i)^2 + Lkd1(i)*Lkd2(i)*Lmd(i)^2 + Lfd(i)*Lmd(i)^2*Lssd(i) + Lkd2(i)*Lmd(i)^2*Lssd(i) - Lfd(i)*Lkd1(i)*Lkd2(i)*Lssd(i))),  + 0,  + 0,  + 0, ; (0 - (Lfd(i)*Lmd(i)^2 + Lkd1(i)*Lmd(i)^2 - Lmd(i)^3 - Lfd(i)*Lkd1(i)*Lmd(i))/(2*Lmd(i)^4 - Lkd1(i)*Lmd(i)^3 - 2*Lkd2(i)*Lmd(i)^3 - Lmd(i)^3*Lssd(i) - 2*Lfd(i)*Lmd(i)^3 + Lfd(i)*Lkd1(i)*Lmd(i)^2 + Lfd(i)*Lkd2(i)*Lmd(i)^2 + Lkd1(i)*Lkd2(i)*Lmd(i)^2 + Lfd(i)*Lmd(i)^2*Lssd(i) + Lkd2(i)*Lmd(i)^2*Lssd(i) - Lfd(i)*Lkd1(i)*Lkd2(i)*Lssd(i))),  + 0,  + (0 - (Lkd1(i)*Lmd(i)^2 + Lmd(i)^2*Lssd(i) - Lmd(i)^3 - Lkd1(i)*Lmd(i)*Lssd(i))/(2*Lmd(i)^4 - Lkd1(i)*Lmd(i)^3 - 2*Lkd2(i)*Lmd(i)^3 - Lmd(i)^3*Lssd(i) - 2*Lfd(i)*Lmd(i)^3 + Lfd(i)*Lkd1(i)*Lmd(i)^2 + Lfd(i)*Lkd2(i)*Lmd(i)^2 + Lkd1(i)*Lkd2(i)*Lmd(i)^2 + Lfd(i)*Lmd(i)^2*Lssd(i) + Lkd2(i)*Lmd(i)^2*Lssd(i) - Lfd(i)*Lkd1(i)*Lkd2(i)*Lssd(i))),  + (0 - (Lfd(i)*Lmd(i)^2 + Lmd(i)^2*Lssd(i) - Lmd(i)^3 - Lfd(i)*Lmd(i)*Lssd(i))/(2*Lmd(i)^4 - Lkd1(i)*Lmd(i)^3 - 2*Lkd2(i)*Lmd(i)^3 - Lmd(i)^3*Lssd(i) - 2*Lfd(i)*Lmd(i)^3 + Lfd(i)*Lkd1(i)*Lmd(i)^2 + Lfd(i)*Lkd2(i)*Lmd(i)^2 + Lkd1(i)*Lkd2(i)*Lmd(i)^2 + Lfd(i)*Lmd(i)^2*Lssd(i) + Lkd2(i)*Lmd(i)^2*Lssd(i) - Lfd(i)*Lkd1(i)*Lkd2(i)*Lssd(i))),  + (0 + (Lfd(i)*Lmd(i)^2 + Lkd1(i)*Lmd(i)^2 + Lmd(i)^2*Lssd(i) - 2*Lmd(i)^3 - Lfd(i)*Lkd1(i)*Lssd(i))/(2*Lmd(i)^4 - Lkd1(i)*Lmd(i)^3 - 2*Lkd2(i)*Lmd(i)^3 - Lmd(i)^3*Lssd(i) - 2*Lfd(i)*Lmd(i)^3 + Lfd(i)*Lkd1(i)*Lmd(i)^2 + Lfd(i)*Lkd2(i)*Lmd(i)^2 + Lkd1(i)*Lkd2(i)*Lmd(i)^2 + Lfd(i)*Lmd(i)^2*Lssd(i) + Lkd2(i)*Lmd(i)^2*Lssd(i) - Lfd(i)*Lkd1(i)*Lkd2(i)*Lssd(i))),  + 0,  + 0,  + 0, ; 0,  + (0 - (Lkq2(i)*Lmq(i)^2 + Lkq3(i)*Lmq(i)^2 - Lmq(i)^3 - Lkq2(i)*Lkq3(i)*Lmq(i))/(3*Lmq(i)^4 - 2*Lkq2(i)*Lmq(i)^3 - 2*Lkq3(i)*Lmq(i)^3 - 2*Lmq(i)^3*Lssq(i) - 2*Lkq1(i)*Lmq(i)^3 + Lkq1(i)*Lkq2(i)*Lmq(i)^2 + Lkq1(i)*Lkq3(i)*Lmq(i)^2 + Lkq2(i)*Lkq3(i)*Lmq(i)^2 + Lkq1(i)*Lmq(i)^2*Lssq(i) + Lkq2(i)*Lmq(i)^2*Lssq(i) + Lkq3(i)*Lmq(i)^2*Lssq(i) - Lkq1(i)*Lkq2(i)*Lkq3(i)*Lssq(i))),  + 0,  + 0,  + 0,  + (0 - (Lmq(i)^2*Lssq(i) + Lkq2(i)*Lkq3(i)*Lssq(i) - Lkq2(i)*Lmq(i)*Lssq(i) - Lkq3(i)*Lmq(i)*Lssq(i))/(3*Lmq(i)^4 - 2*Lkq2(i)*Lmq(i)^3 - 2*Lkq3(i)*Lmq(i)^3 - 2*Lmq(i)^3*Lssq(i) - 2*Lkq1(i)*Lmq(i)^3 + Lkq1(i)*Lkq2(i)*Lmq(i)^2 + Lkq1(i)*Lkq3(i)*Lmq(i)^2 + Lkq2(i)*Lkq3(i)*Lmq(i)^2 + Lkq1(i)*Lmq(i)^2*Lssq(i) + Lkq2(i)*Lmq(i)^2*Lssq(i) + Lkq3(i)*Lmq(i)^2*Lssq(i) - Lkq1(i)*Lkq2(i)*Lkq3(i)*Lssq(i))),  + 0,  + 0, ; 0,  + (0 + (Lmq(i)*(Lkq1(i) - Lmq(i))*(Lkq3(i) - Lmq(i)))/(3*Lmq(i)^4 - 2*Lkq2(i)*Lmq(i)^3 - 2*Lkq3(i)*Lmq(i)^3 - 2*Lmq(i)^3*Lssq(i) - 2*Lkq1(i)*Lmq(i)^3 + Lkq1(i)*Lkq2(i)*Lmq(i)^2 + Lkq1(i)*Lkq3(i)*Lmq(i)^2 + Lkq2(i)*Lkq3(i)*Lmq(i)^2 + Lkq1(i)*Lmq(i)^2*Lssq(i) + Lkq2(i)*Lmq(i)^2*Lssq(i) + Lkq3(i)*Lmq(i)^2*Lssq(i) - Lkq1(i)*Lkq2(i)*Lkq3(i)*Lssq(i))),  + 0,  + 0,  + 0,  + (0 - (Lssq(i)*(Lkq1(i) - Lmq(i))*(Lkq3(i) - Lmq(i)))/(3*Lmq(i)^4 - 2*Lkq2(i)*Lmq(i)^3 - 2*Lkq3(i)*Lmq(i)^3 - 2*Lmq(i)^3*Lssq(i) - 2*Lkq1(i)*Lmq(i)^3 + Lkq1(i)*Lkq2(i)*Lmq(i)^2 + Lkq1(i)*Lkq3(i)*Lmq(i)^2 + Lkq2(i)*Lkq3(i)*Lmq(i)^2 + Lkq1(i)*Lmq(i)^2*Lssq(i) + Lkq2(i)*Lmq(i)^2*Lssq(i) + Lkq3(i)*Lmq(i)^2*Lssq(i) - Lkq1(i)*Lkq2(i)*Lkq3(i)*Lssq(i))),  + 0,  + 0, ; 0,  + (0 + (Lmq(i)*(Lkq1(i) - Lmq(i))*(Lkq2(i) - Lmq(i)))/(3*Lmq(i)^4 - 2*Lkq2(i)*Lmq(i)^3 - 2*Lkq3(i)*Lmq(i)^3 - 2*Lmq(i)^3*Lssq(i) - 2*Lkq1(i)*Lmq(i)^3 + Lkq1(i)*Lkq2(i)*Lmq(i)^2 + Lkq1(i)*Lkq3(i)*Lmq(i)^2 + Lkq2(i)*Lkq3(i)*Lmq(i)^2 + Lkq1(i)*Lmq(i)^2*Lssq(i) + Lkq2(i)*Lmq(i)^2*Lssq(i) + Lkq3(i)*Lmq(i)^2*Lssq(i) - Lkq1(i)*Lkq2(i)*Lkq3(i)*Lssq(i))),  + 0,  + 0,  + 0,  + (0 - (Lssq(i)*(Lkq1(i) - Lmq(i))*(Lkq2(i) - Lmq(i)))/(3*Lmq(i)^4 - 2*Lkq2(i)*Lmq(i)^3 - 2*Lkq3(i)*Lmq(i)^3 - 2*Lmq(i)^3*Lssq(i) - 2*Lkq1(i)*Lmq(i)^3 + Lkq1(i)*Lkq2(i)*Lmq(i)^2 + Lkq1(i)*Lkq3(i)*Lmq(i)^2 + Lkq2(i)*Lkq3(i)*Lmq(i)^2 + Lkq1(i)*Lmq(i)^2*Lssq(i) + Lkq2(i)*Lmq(i)^2*Lssq(i) + Lkq3(i)*Lmq(i)^2*Lssq(i) - Lkq1(i)*Lkq2(i)*Lkq3(i)*Lssq(i))),  + 0,  + 0, ];
      |     end
  isd : Outport
  isq : Outport  Port=2
  psi : Outport  Port=3
  ifd : Outport  Port=4

== system VFlexP/Grid/Generators/MGES/For Each Subsystem ==
  In1 : Inport  Partition=on  PartitionDimension=1  PartitionWidth=1  PartitionOffset=0
  For Each : ForEach  DisableCoverage=on
  State-Space : StateSpace  A=[]  B=[]  C=[]  D=block_toM  InitialCondition=0  ParameterTunability=Optimized
  Transpose : Math  Operator=transpose
  Transpose1 : Math  Operator=transpose
  Out1 : Outport  ConcatenationDimension=1
  wires:
  Transpose1/1 -> Out1/1
  In1/1 -> Transpose/1
  Transpose/1 -> State-Space/1
  State-Space/1 -> Transpose1/1

== system VFlexP/Grid/Generators/MGES/LPF1 ==
  in : Inport
  Gain : Gain  Gain=1./T_s
  Sum4 : Sum  Inputs=|+-
  x_a : Integrator  InitialConditionSource=external  InitialCondition=Grid_op_MGES.op.States(16).x'
  out : Outport
  wires:
  Gain/1 -> x_a/1
  Sum4/1 -> Gain/1
  in/1 -> x_a/2, Sum4/1
  x_a/1 -> out/1, Sum4/2

== system VFlexP/Grid/Generators/MGES/LPF2 ==
  in : Inport
  Gain : Gain  Gain=1./T_s
  Sum4 : Sum  Inputs=|+-
  x_a : Integrator  InitialConditionSource=external  InitialCondition=Grid_op_MGES.op.States(17).x'
  out : Outport
  wires:
  Gain/1 -> x_a/1
  Sum4/1 -> Gain/1
  in/1 -> x_a/2, Sum4/1
  x_a/1 -> out/1, Sum4/2

== system VFlexP/Grid/Generators/MGES/LPF3 ==
  in : Inport
  Gain : Gain  Gain=1./T_s
  Sum4 : Sum  Inputs=|+-
  x_a : Integrator  InitialConditionSource=external  InitialCondition=Grid_op_MGES.op.States(18).x'
  out : Outport
  wires:
  Gain/1 -> x_a/1
  Sum4/1 -> Gain/1
  in/1 -> x_a/2, Sum4/1
  x_a/1 -> out/1, Sum4/2

== system VFlexP/Grid/Generators/MGES/LPF4 ==
  in : Inport
  Gain : Gain  Gain=1./T_s
  Sum4 : Sum  Inputs=|+-
  x_a : Integrator  InitialCondition=Grid_op_SG.op.States(10).x'
  out : Outport
  wires:
  x_a/1 -> Sum4/2, out/1
  in/1 -> Sum4/1
  Sum4/1 -> Gain/1
  Gain/1 -> x_a/1

== system VFlexP/Grid/Generators/MGES/LPF5 ==
  in : Inport
  Gain : Gain  Gain=1./T_s
  Sum4 : Sum  Inputs=|+-
  x_a : Integrator  InitialCondition=Grid_op_SG.op.States(11).x'
  out : Outport
  wires:
  Gain/1 -> x_a/1
  Sum4/1 -> Gain/1
  in/1 -> Sum4/1
  x_a/1 -> out/1, Sum4/2

== system VFlexP/Grid/Generators/MGES/LPF6 ==
  in : Inport
  Gain : Gain  Gain=1./T_s
  Sum4 : Sum  Inputs=|+-
  x_a : Integrator  InitialConditionSource=external  InitialCondition=Grid_op_MGES.op.States(19).x'
  out : Outport
  wires:
  Gain/1 -> x_a/1
  Sum4/1 -> Gain/1
  in/1 -> x_a/2, Sum4/1
  x_a/1 -> out/1, Sum4/2

== system VFlexP/Grid/Generators/MGES/LeadLag ==
  In1 : Inport
  AVR_LeadLag : Subsystem  mask{T_2=T_2(T_1~=0), T_1=T_1(T_1~=0)}
      mask help:
      | Transfer function:
      |
      |   1 + sT_2
      | ---------------
      |   1 + sT_1
  Assignment1 : Assignment  DiagnosticForDimensions=Warning  IndexOptions=Index vector (dialog)  Indices=find(T_1~=0)  OutputSizes=1
  Selector10 : Selector  InputPortWidth=length(block_buses)  IndexOptions=Index vector (dialog)  Indices=find(T_1~=0)  OutputSizes=1
  Out1 : Outport
  wires:
  AVR_LeadLag/1(Out1) -> Assignment1/2
  Selector10/1 -> AVR_LeadLag/1(In1)
  Assignment1/1 -> Out1/1
  In1/1 -> Assignment1/1, Selector10/1

== system VFlexP/Grid/Generators/MGES/LeadLag1 ==
  In1 : Inport
  Gain : Gain  Gain=1./T_1
  Gain2 : Gain  Gain=T_2./T_1
  Sum : Sum  Inputs=|+-
  Sum1 : Sum  Inputs=++|
  x_f : Integrator  InitialConditionSource=external  InitialCondition=Grid_op_MGES.op.States(21).x'
  Out1 : Outport
  wires:
  x_f/1 -> Sum1/2, Sum/2
  Gain/1 -> x_f/1
  Sum/1 -> Gain/1, Gain2/1
  Gain2/1 -> Sum1/1
  Sum1/1 -> Out1/1
  In1/1 -> x_f/2, Sum/1

== system VFlexP/Grid/Generators/MGES/LeadLag2 ==
  In1 : Inport
  Gain : Gain  Gain=1./T_1
  Gain2 : Gain  Gain=T_2./T_1
  Sum : Sum  Inputs=|+-
  Sum1 : Sum  Inputs=++|
  x_f : Integrator  InitialConditionSource=external  InitialCondition=Grid_op_MGES.op.States(22).x'
  Out1 : Outport
  wires:
  In1/1 -> Sum/1, x_f/2
  Sum1/1 -> Out1/1
  Gain2/1 -> Sum1/1
  Sum/1 -> Gain2/1, Gain/1
  Gain/1 -> x_f/1
  x_f/1 -> Sum/2, Sum1/2

== system VFlexP/Grid/Generators/MGES/PI1 ==
  In1 : Inport
  Gain1 : Gain  Gain=K_IM ~= 0
  Gain4 : Gain  Gain=K_PM
  Gain5 : Gain  Gain=K_IM
  Integrator : Integrator  InitialCondition=Grid_op_MGES.op.States(23).x'
  Sum7 : Sum  Inputs=|++
  vfd : Outport
  wires:
  Integrator/1 -> Gain1/1
  Gain4/1 -> Sum7/1
  Sum7/1 -> vfd/1
  In1/1 -> Gain4/1, Gain5/1
  Gain5/1 -> Integrator/1
  Gain1/1 -> Sum7/2

== system VFlexP/Grid/Generators/MGES/PI2 ==
  In1 : Inport
  Gain1 : Gain  Gain=K_IR ~= 0
  Gain4 : Gain  Gain=K_PR
  Gain5 : Gain  Gain=K_IR
  Integrator : Integrator  InitialCondition=Grid_op_MGES.op.States(24).x'
  Sum7 : Sum  Inputs=|++
  Out1 : Outport
  wires:
  Integrator/1 -> Gain1/1
  Gain4/1 -> Sum7/1
  Sum7/1 -> Out1/1
  In1/1 -> Gain4/1, Gain5/1
  Gain5/1 -> Integrator/1
  Gain1/1 -> Sum7/2

== system VFlexP/Grid/Generators/MGES/Reference frame transform1 ==
  in_d : Inport
  theta : Inport  Port=2
  in_q : Inport  Port=3
  Complex to Real-Imag : ComplexToRealImag
  Cos : Trigonometry  SCDEnableBlockLinearizationSpecification=on  Operator=cos
  Product : Product
  Real-Imag to Complex : RealImagToComplex
  Real-Imag to Complex1 : RealImagToComplex
  Sin : Trigonometry  SCDEnableBlockLinearizationSpecification=on
  out_d : Outport
  out_q : Outport  Port=2
  wires:
  in_d/1 -> Real-Imag to Complex/1
  in_q/1 -> Real-Imag to Complex/2
  Complex to Real-Imag/1 -> out_d/1
  Sin/1 -> Real-Imag to Complex1/2
  Cos/1 -> Real-Imag to Complex1/1
  theta/1 -> Cos/1, Sin/1
  Product/1 -> Complex to Real-Imag/1
  Real-Imag to Complex/1 -> Product/2
  Real-Imag to Complex1/1 -> Product/1
  Complex to Real-Imag/2 -> out_q/1

== system VFlexP/Grid/Generators/MGES/Reference frame transform3 ==
  in_d : Inport
  theta : Inport  Port=2
  in_q : Inport  Port=3
  Complex to Real-Imag : ComplexToRealImag
  Cos : Trigonometry  SCDEnableBlockLinearizationSpecification=on  Operator=cos
  Product : Product
  Real-Imag to Complex : RealImagToComplex
  Real-Imag to Complex1 : RealImagToComplex
  Sin : Trigonometry  SCDEnableBlockLinearizationSpecification=on
  out_d : Outport
  out_q : Outport  Port=2
  wires:
  Complex to Real-Imag/2 -> out_q/1
  Real-Imag to Complex1/1 -> Product/1
  Real-Imag to Complex/1 -> Product/2
  Product/1 -> Complex to Real-Imag/1
  theta/1 -> Sin/1, Cos/1
  Cos/1 -> Real-Imag to Complex1/1
  Sin/1 -> Real-Imag to Complex1/2
  Complex to Real-Imag/1 -> out_d/1
  in_q/1 -> Real-Imag to Complex/2
  in_d/1 -> Real-Imag to Complex/1

== system VFlexP/Grid/Generators/MGES/Rotor axis ==
  te : Inport
  tm : Inport  Port=2
  Gain : Gain  Gain=1/2./H
  Gain1 : Gain  Gain=D
  Sum1 : Sum  Inputs=+|-|-  InputSameDT=on  SaturateOnIntegerOverflow=on  OutDataTypeStr=Inherit: Same as first input
  \omega_r : Integrator  InitialCondition=Grid_op_MGES.op.States(25).x'  UpperSaturationLimit=2*pi  LowerSaturationLimit=0
  wr : Outport  VectorParamsAs1DForOutWhenUnconnected=off
  wires:
  tm/1 -> Sum1/1
  \omega_r/1 -> wr/1, Gain1/1
  te/1 -> Sum1/2
  Sum1/1 -> Gain/1
  Gain/1 -> \omega_r/1
  Gain1/1 -> Sum1/3

== system VFlexP/Grid/Generators/MGES/Subsystem ==
  in : Inport
  LPF1 : Subsystem  mask{T_s=T_9}
      mask prompts: T_s "Filter time constant"
  LPF2 : Subsystem  mask{T_s=T_9}
      mask prompts: T_s "Filter time constant"
  LPF3 : Subsystem  mask{T_s=T_9}
      mask prompts: T_s "Filter time constant"
  LPF4 : Subsystem  mask{T_s=T_9}
      mask prompts: T_s "Filter time constant"
  LPF7 : Subsystem  mask{T_s=T_9}
      mask prompts: T_s "Filter time constant"
  out : Outport
  wires:
  LPF2/1(out) -> LPF3/1(in)
  LPF3/1(out) -> LPF4/1(in)
  LPF7/1(out) -> LPF1/1(in)
  LPF4/1(out) -> out/1
  LPF1/1(out) -> LPF2/1(in)
  in/1 -> LPF7/1(in)

== system VFlexP/Grid/Generators/MGES/Subsystem1 ==
  vt : Inport
  ifd : Inport  Port=2
  Assignment1 : Assignment  DiagnosticForDimensions=Warning  IndexOptions=Index vector (dialog)  Indices=find(K_P~=0)  OutputSizes=1
  Divide1 : Product  Inputs=*/
  Gain11 : Gain  Gain=K_C(K_P~=0)
  Gain12 : Gain  Gain=K_P(K_P~=0)
  MATLAB Function : MATLAB Function  TreatAsAtomicUnit=on
  One : Constant  Value=ones(1, length(block_buses))  VectorParams1D=off  OutDataTypeStr=Inherit: Inherit via back propagation
  Product5 : Product
  Selector1 : Selector  InputPortWidth=length(block_buses)  IndexOptions=Index vector (dialog)  Indices=find(K_P~=0)  OutputSizes=1
  Selector9 : Selector  InputPortWidth=length(block_buses)  IndexOptions=Index vector (dialog)  Indices=find(K_P~=0)  OutputSizes=1
  V_B : Outport
  wires:
  Product5/1 -> Assignment1/2
  One/1 -> Assignment1/1
  vt/1 -> Selector9/1
  Assignment1/1 -> V_B/1
  Selector9/1 -> Gain12/1
  Gain11/1 -> Divide1/1
  MATLAB Function/1(F_EX) -> Product5/1
  Gain12/1 -> Divide1/2, Product5/2
  ifd/1 -> Selector1/1
  Selector1/1 -> Gain11/1
  Divide1/1 -> MATLAB Function/1(I_N)

== system VFlexP/Grid/Generators/MGES/Subsystem4 ==
  In1 : Inport
  Gain : Gain  Gain=1./T_1
  Gain2 : Gain  Gain=T_2./T_1
  Sum : Sum  Inputs=|+-
  Sum1 : Sum  Inputs=++|
  x_f : Integrator  InitialCondition=Grid_op_MGES.op.States(21).x'
  Out1 : Outport
  wires:
  x_f/1 -> Sum1/2, Sum/2
  Gain/1 -> x_f/1
  Sum/1 -> Gain/1, Gain2/1
  Gain2/1 -> Sum1/1
  Sum1/1 -> Out1/1
  In1/1 -> Sum/1

== system VFlexP/Grid/Generators/MGES/Torque ==
  psi : Inport
  isd : Inport  Port=2
  isq : Inport  Port=3
  Product1 : Product
  Product2 : Product
  Selector : Selector  NumberOfDimensions=2  InputPortWidth=9  IndexOptions=Index vector (dialog),Select all  Indices=[1],1  OutputSizes=1,1
  Selector1 : Selector  NumberOfDimensions=2  InputPortWidth=9  IndexOptions=Index vector (dialog),Select all  Indices=[2],1  OutputSizes=1,1
  Sum : Sum  Inputs=+||-
  te : Outport  VectorParamsAs1DForOutWhenUnconnected=off
  wires:
  Product1/1 -> Sum/1
  Sum/1 -> te/1
  Selector/1 -> Product1/1  "psistatordq"
  psi/1 -> Selector1/1, Selector/1
  Product2/1 -> Sum/2
  isq/1 -> Product1/2
  isd/1 -> Product2/1
  Selector1/1 -> Product2/2  "psistatordq"

== system VFlexP/Grid/Generators/MGES/WOF_d ==
  In1 : Inport
  Gain : Gain  Gain=1/T_w1
  I : Integrator  InitialConditionSource=external  InitialCondition=Grid_op_MGES.op.States(31).x'
  Sum : Sum  Inputs=+-|
  Sum4 : Sum  Inputs=|+-
  Out1 : Outport
  wires:
  Sum/1 -> Out1/1
  I/1 -> Sum/2, Sum4/2
  In1/1 -> Sum4/1, Sum/1, I/2
  Sum4/1 -> Gain/1
  Gain/1 -> I/1

== system VFlexP/Grid/Generators/MGES/WOF_d1 ==
  In1 : Inport
  Gain : Gain  Gain=1/T_w2
  I : Integrator  InitialConditionSource=external  InitialCondition=Grid_op_MGES.op.States(32).x'
  Sum : Sum  Inputs=+-|
  Sum4 : Sum  Inputs=|+-
  Out1 : Outport
  wires:
  Sum/1 -> Out1/1
  I/1 -> Sum/2, Sum4/2
  In1/1 -> Sum4/1, Sum/1, I/2
  Sum4/1 -> Gain/1
  Gain/1 -> I/1

== system VFlexP/Grid/Generators/MGES/connect ==
  id : Inport
  iq : Inport  Port=2
  connect : Inport  Port=3
  Switch : Switch  Criteria=u2 > Threshold  ZeroCross=off  SaturateOnIntegerOverflow=off  InputSameDT=off
  Switch1 : Switch  Criteria=u2 > Threshold  ZeroCross=off  SaturateOnIntegerOverflow=off  InputSameDT=off
  Zero1 : Constant  Value=0  VectorParams1D=off  OutDataTypeStr=Inherit: Inherit via back propagation
  Zero2 : Constant  Value=0  VectorParams1D=off  OutDataTypeStr=Inherit: Inherit via back propagation
  id_real : Outport
  iq_real : Outport  Port=2
  connected : Outport  Port=3  OutDataTypeStr=boolean
  wires:
  Switch/1 -> id_real/1
  Zero1/1 -> Switch/3
  id/1 -> Switch/1
  connect/1 -> connected/1, Switch1/2, Switch/2
  Switch1/1 -> iq_real/1
  iq/1 -> Switch1/1
  Zero2/1 -> Switch1/3

== system VFlexP/Grid/Generators/MGES/trim_output ==
  id : Inport
  iq : Inport  Port=2
  vd : Inport  Port=3
  vq : Inport  Port=4
  Out1 : Outport
  Out2 : Outport  Port=2
  Out3 : Outport  Port=3
  Out4 : Outport  Port=4
  wires:
  id/1 -> Out1/1
  vq/1 -> Out4/1
  vd/1 -> Out3/1
  iq/1 -> Out2/1
